simulink model "CEGR_TestBench_10kW_v01_pO2_DQ60"  (R2025b)
settings: Solver=FixedStepDiscrete  StartTime=0.0  StopTime=120  FixedStep=0.1  RelTol=1e-3
InitFcn:
  | modelFile=get_param(bdroot,'FileName'); projectDir=fileparts(fileparts(modelFile)); addpath(fullfile(projectDir,'02_脚本')); prepare_testbench_10kw_v01_model_run(bdroot);
model workspace (MAT data in the model file):
  BenchAirParam_v1 = [96485.33212; 0.031998; 0.0280134; 0.01801528; 112.325; 58.9; 0.8; 0.2095; 0.7905; 16; 2; 0.00428414; 141.325; 58.9; 0.8]
  BenchConditionerParam_v1 = [0.031998; 0.0280134; 0.01801528; 101.325; 58.9; 141.325]
  CompressorParam_v2 = [8.314462618; 0.031998; 0.0280134; 0.01801528; 1.4; 1005; 0.62; 4000; 3000; 4000; 5000; 6000; 7000; 8000; 80; 170; 420; 590; 780; 960; 120; 220; 500; 650; 830; 1030; 160; 300; 580; 690; 890; 1070; 210; 380; 660; 760; 940; 1120; 300; 500; 720; 820; 990; 1160; 450; 590; 760; 880; 1040; 1200; 29; 39.5; 36.5; 40; 44.5; 43.5; 25; 33; 26; 33; 35; 32; 22; 27; 16; 27.5; 28; 25; 16; 18.5; 10.5; 19.5; 20.5; 18; 9; 9; 6; 13; 15; 15; 2.5; 4; 3; 8; 7; 6.5]
  EGRInitialNode_v2 = [0; 0; 0; 0; 56; 133.825; 0]
  EnvParam_v2 = [96485.33212; 0.031998; 0.0280134; 0.01801528; 101.325; 25; 0.5; 0.2095; 0.7905; 16; 2]
  HumidifierParam_v2 = [0.031998; 0.0280134; 0.01801528; 101.325; 55; 0.47854; 0.0983333333333; 0.37998; 0.5825; 9.51831; 11.4663; 0.578752; 40; 5e-05; 1e-09; 0.06; 0.06; 80]
  I_stack_cmd_A = 38
  IntercoolerParam_v2 = [0.031998; 0.0280134; 0.01801528; 101.325; 55; 8]
  P_v2.rootDir = 'E:\Codex\agentwork_pemfc_cEGR_0519\01_自吸方案\01_车载系统_10kW_GZS60_v3'
  P_v2.inputDir = 'E:\Codex\agentwork_pemfc_cEGR_0519\01_自吸方案\01_车载系统_10kW_GZS60_v3\00_输入参数'
  P_v2.modelName = 'CEGR_Vehicle_10kW_GZS60_v03_stage1_pressurefix'
  P_v2.modelFile = 'E:\Codex\agentwork_pemfc_cEGR_0519\01_自吸方案\01_车载系统_10kW_GZS60_v3\01_模型\CEGR_Vehicle_10kW_GZS60_v03_stage1_pressurefix.slx'
  P_v2.calibration_baseline = "stage1_pressurefix_no_egr"
  P_v2.stopTime_s = 120
  P_v2.dt_s = 0.1
  P_v2.R_J_molK = 8.314462618
  P_v2.F_C_mol = 96485.33212
  P_v2.M_O2_kg_mol = 0.031998
  P_v2.M_N2_kg_mol = 0.0280134
  P_v2.M_H2O_kg_mol = 0.01801528
  P_v2.M_H2_kg_mol = 0.00201588
  P_v2.p_amb_kPa = 101.325
  P_v2.T_amb_C = 25
  P_v2.RH_amb = 0.5
  P_v2.xO2_dry = 0.2095
  P_v2.xN2_dry = 0.7905
  P_v2.N_cell = 16
  P_v2.A_cell_cm2 = 380
  P_v2.I_stack_default_A = 120
  P_v2.oxygen_stoich = 2
  P_v2.anode_stoich = 1.35
  P_v2.RH_an_in = 0.3
  P_v2.compressor_dp_kPa = 55
  P_v2.compressor_dT_C = 35
  P_v2.intercooler_T_C = 55
  P_v2.intercooler_dp_kPa = 8
  P_v2.p_cathode_back_kPa = 128
  P_v2.p_anode_back_kPa = 85
  P_v2.p_anode_in_kPa = 140
  P_v2.K_ca_in_kg_s_kPa = 0.0003
  P_v2.hum_NTU_ref = 0.47854
  P_v2.hum_m_ref_kg_s = 0.0983333333333
  P_v2.hum_flow_exp = 0.37998
  P_v2.hum_heat_eff = 0.5825
  P_v2.hum_dry_dp_ref_kPa = 9.51831
  P_v2.hum_wet_dp_ref_kPa = 11.4663
  P_v2.hum_dp_exp = 0.578752
  P_v2.hum_mem_area_m2 = 40
  P_v2.hum_mem_thickness_m = 5e-05
  P_v2.hum_mem_D_eff_m2_s = 1e-09
  P_v2.hum_beta_wet_m_s = 0.06
  P_v2.hum_beta_dry_m_s = 0.06
  P_v2.hum_UA_W_K = 80
  P_v2.V_ca_m3 = 0.0002
  P_v2.V_an_m3 = 0.00015
  P_v2.K_ca_out_kg_s_kPa = 0.00012
  P_v2.K_an_out_kg_s_kPa = 6.67e-06
  P_v2.K_liq_carry_1_s = 0.08
  P_v2.C_stack_J_K = 45000
  P_v2.h_cool_W_K = 836
  P_v2.T_cool_C = 62
  P_v2.h_amb_W_K = 9
  P_v2.coolant_flow_L_min = 6
  P_v2.coolant_rho_kg_L = 1
  P_v2.coolant_cp_J_kgK = 4180
  P_v2.cool_flow_curve_enabled = 1
  P_v2.cool_flow_curve_L_min = [5.5 6 6.5 7.5 9.1 10 11.1 11.5 0 0 0 0 0]
  P_v2.cool_flow_curve_h_W_K = [836 836 905.666666667 1045 1267.93333333 1393.33333333 1546.6 1602.33333333 0 0 0 0 0]
  P_v2.k_mem_water_kg_s = 0.00012
  P_v2.E_nernst_ref_V = 1.229
  P_v2.E_nernst_temp_coeff_V_K = 0.00085
  P_v2.book_theta1 = 0.304017191982
  P_v2.book_theta2 = 2.2530615997e-05
  P_v2.book_theta3 = -2.43220427369e-40
  P_v2.book_theta4 = 6.6267870644e-05
  P_v2.book_theta5 = 0.0455473243079
  P_v2.book_theta6 = 6.57684656899e-05
  P_v2.book_theta7 = -1.52874181623
  P_v2.book_theta8 = 9.63813640803e-05
  P_v2.book_theta9 = 2.42869264824e-06
  P_v2.book_theta10 = 0.00979289103499
  P_v2.membraneThickness_cm = 0.005
  P_v2.thermoneutralVoltage_V = 1.254
  P_v2.LHV_H2_J_mol = 241800
  P_v2.stack_m_act_O2 = 0.65
  P_v2.stack_m_lim_O2 = 1.2
  P_v2.stack_i_lim_ref_A_cm2 = 1.2
  P_v2.stack_lambda_O2_half = 1.2
  P_v2.egr_fraction_default = 0.4
  P_v2.EnvParam = [96485.33212; 0.031998; 0.0280134; 0.01801528; 101.325; 25; 0.5; 0.2095; 0.7905; 16; 2]
  P_v2.CompressorParam = [55; 35]
  P_v2.IntercoolerParam = [0.031998; 0.0280134; 0.01801528; 101.325; 55; 8]
  P_v2.HumidifierParam = [0.031998; 0.0280134; 0.01801528; 101.325; 55; 0.47854; 0.0983333333333; 0.37998; 0.5825; 9.51831; 11.4663; 0.578752; 40; 5e-05; 1e-09; 0.06; 0.06; 80]
  P_v2.StackParam = [8.314462618; 96485.33212; 0.031998; 0.0280134; 0.01801528; 0.00201588; 101.325; 25; 16; 380; 0.0002; 0.00015; 0.00012; 6.67e-06; 128; 85; 0.08; 45000; 836; 62; 9; 1.229; 0.00085; 0.304017191982; 2.2530615997e-05; -2.43220427369e-40; 6.6267870644e-05; 0.005; 9.63813640803e-05; 2.42869264824e-06; 0.00979289103499; 1.254; 1.35; 0.3; 0.1; 0.00012; 140; 0.0003; 0.65; 1.2; 1.2; 1.2; 241800; 6; 1; 5.5; 6; 6.5; 7.5; 9.1; 10; 11.1; 11.5; 0; 0; 0; 0; 0; 836; 836; 905.666666667; 1045; 1267.93333333; 1393.33333333; 1546.6; 1602.33333333; 0; 0; 0; 0; 0; 0.0455473243079; 6.57684656899e-05; -1.52874181623]
  P_v2.egr_initial_node = [0; 0; 0; 0; 25; 101.325; 0]
  P_v2.wet_initial_node = [0; 0; 0; 0; 70; 128; 0]
  P_v2.stack_initial_state = [5.69048472088e-05; 0.000189310998745; 3.20381510039e-05; 0; 1.39815625735e-05; 7.2204543855e-06; 0; 65]
  P_v2.stack_initial_state_audit = [5.69048472088e-05; 0.000189310998745; 3.20381510039e-05; 1.39815625735e-05; 7.2204543855e-06; 65]
  StackInitialStateAudit_v3 = [5.69048472088e-05; 0.000189310998745; 3.20381510039e-05; 1.39815625735e-05; 7.2204543855e-06; 65]
  StackInitialState_v2 = [5.89666776843e-05; 0.000206495047021; 1.97861723777e-05; 1.38831382347e-05; 5.56486098123e-06; 58.9]
  StackParam_v2 = [8.314462618; 96485.33212; 0.031998; 0.0280134; 0.01801528; 0.00201588; 101.325; 25; 16; 380; 0.0002; 0.00015; 0.00012; 6.67e-06; 133.825; 144.725; 0.08; 45000; 1156.46666667; 61.6; 9; 1.229; 0.00085; 0.304017191982; 2.2530615997e-05; -2.43220427369e-40; 6.6267870644e-05; 0.005; 9.63813640803e-05; 2.42869264824e-06; 0.00979289103499; 1.254; 5; 0.3; 0.1; 0.00012; 149.125; 0.000571218666667; 0.65; 1.2; 1.2; 1.2; 241800; 5.5; 1; 6; 6.5; 7.5; 9.1; 10; 11.1; 11.5; 0; 0; 0; 0; 0; 0; 1156.46666667; 1156.46666667; 1285.06756757; 1415.36744186; 1614.22764228; 1614.22764228; 1637.16666667; 0; 0; 0; 0; 0; 0; 0.0455473243079; 6.57684656899e-05; -1.52874181623]
  WetInitialNode_v2 = [0; 0; 0; 0; 70; 128; 0]
  egr_fraction_cmd = 0.25
  egr_initial_node = [0; 0; 0; 0; 25; 101.325; 0]
  stack_initial_state_audit = [5.69048472088e-05; 0.000189310998745; 3.20381510039e-05; 1.39815625735e-05; 7.2204543855e-06; 65]
  wet_initial_node = [0; 0; 0; 0; 70; 128; 0]
settings Model: Creator=ADMIN  LastModifiedBy=92465

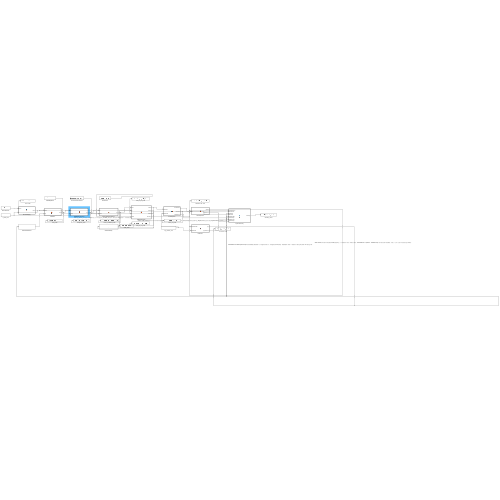
[thumbnail: Simulink's stored preview of the top-level diagram]
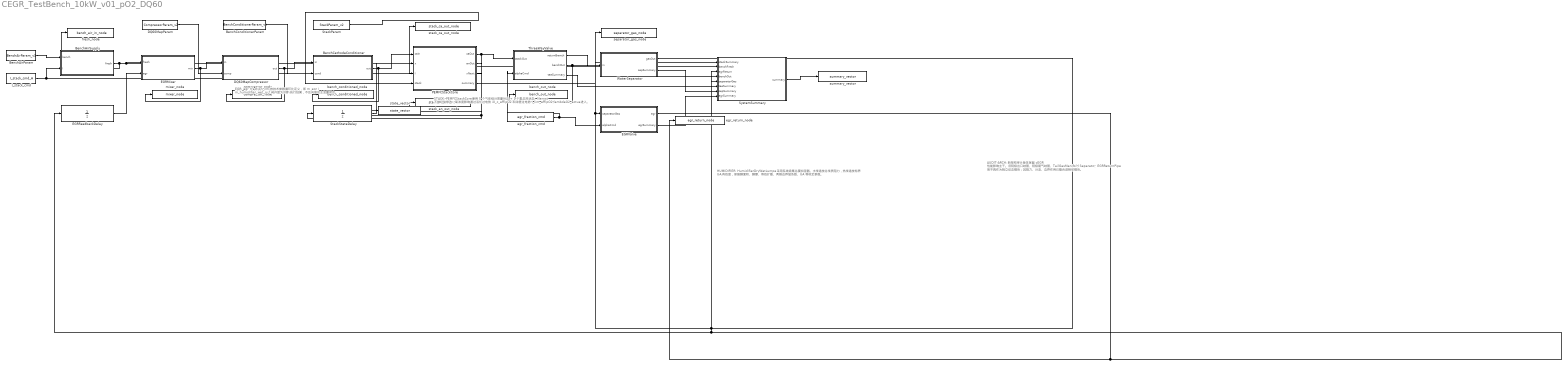
== system CEGR_TestBench_10kW_v01_pO2_DQ60 ==
  note: AUDIT-ARCH: 新架构审计版仅保留 cEGR 性能影响主干。旧阴极出口歧管、阳极尾气歧管、TailGasManifold、Separator、EGRReturnPipe 等不再作为独立动态模块；其阻力、分流、边界作用已整合进相邻模块。
  note: STACK: PEMFCStackCore 使用 5 个气体组分质量状态 + 1 个集总热状态。Nernst 不做经验修改，氧浓度影响通过活化过电势 i0_c_eff(pO2) 和浓差过电势 i_lim_eff(pO2,lambdaO2_actual) 进入。
  note: HUMIDIFIER: HumidifierDryWetLumped 采用系统级集总膜加湿器。水传递按总传质阻力，热传递按有界 UA/有效度，保留膜面积、膜厚、等效扩散、两侧边界层系数、UA 等标定参数。
  note: EGR: egr_fraction_cmd 按技术参数循环比定义，即 m_egr / m_humidifier_wet_out。阀开度为诊断/执行结果，不反向驱动主流量闭合。
  BenchAirParam : Constant  Value=BenchAirParam_v1
  BenchAirSupply : MATLAB Function  TreatAsAtomicUnit=on
  BenchCathodeConditioner : MATLAB Function  TreatAsAtomicUnit=on
  BenchConditionerParam : Constant  Value=BenchConditionerParam_v1
  DQ60MapCompressor : MATLAB Function  TreatAsAtomicUnit=on
  DQ60MapParam : Constant  Value=CompressorParam_v2
  EGRFeedbackDelay : UnitDelay  InitialCondition=EGRInitialNode_v2  SampleTime=-1  HasFrameUpgradeWarning=on
  EGRMixer : MATLAB Function  TreatAsAtomicUnit=on
  EGRValve : MATLAB Function  TreatAsAtomicUnit=on
  I_stack_cmd : Constant  Value=I_stack_cmd_A
  PEMFCStackCore : MATLAB Function  TreatAsAtomicUnit=on
  StackParam : Constant  Value=StackParam_v2
  StackStateDelay : UnitDelay  InitialCondition=StackInitialStateAudit_v3  SampleTime=-1  HasFrameUpgradeWarning=on
  SystemSummary : MATLAB Function  TreatAsAtomicUnit=on
  ThreeWayValve : MATLAB Function  TreatAsAtomicUnit=on
  WaterSeparator : MATLAB Function  TreatAsAtomicUnit=on
  bench_conditioned_node : ToWorkspace  VariableName=bench_conditioned_node  SampleTime=-1
  bench_out_node : ToWorkspace  VariableName=bench_out_node  SampleTime=-1
  compressor_node : ToWorkspace  VariableName=compressor_node  SampleTime=-1
  egr_fraction_cmd : Constant  Value=egr_fraction_cmd
  egr_return_node : ToWorkspace  VariableName=egr_return_node  SampleTime=-1
  fresh_node : ToWorkspace  VariableName=bench_air_in_node  SampleTime=-1
  mixer_node : ToWorkspace  VariableName=mixer_node  SampleTime=-1
  separator_gas_node : ToWorkspace  VariableName=separator_gas_node  SampleTime=-1
  stack_an_out_node : ToWorkspace  VariableName=stack_an_out_node  SampleTime=-1
  stack_ca_out_node : ToWorkspace  VariableName=stack_ca_out_node  SampleTime=-1
  state_vector : ToWorkspace  VariableName=state_vector  SampleTime=-1
  summary_vector : ToWorkspace  VariableName=summary_vector  SampleTime=-1
  wires:
  BenchAirParam/1 -> BenchAirSupply/1(bench)
  I_stack_cmd/1 -> BenchAirSupply/2(I), PEMFCStackCore/3(I)
  BenchAirSupply/1(fresh) -> SystemSummary/2(benchFresh), EGRMixer/1(fresh), fresh_node/1
  EGRFeedbackDelay/1 -> EGRMixer/2(egr)
  EGRMixer/1(mix) -> DQ60MapCompressor/1(in), mixer_node/1
  DQ60MapParam/1 -> DQ60MapCompressor/2(comp)
  DQ60MapCompressor/1(out) -> BenchCathodeConditioner/1(in), compressor_node/1
  BenchConditionerParam/1 -> BenchCathodeConditioner/2(cond)
  BenchCathodeConditioner/1(out) -> bench_conditioned_node/1, PEMFCStackCore/1(caIn)
  StackStateDelay/1 -> PEMFCStackCore/2(x)
  StackParam/1 -> PEMFCStackCore/4(stack)
  PEMFCStackCore/1(caOut) -> ThreeWayValve/1(stackOut), stack_ca_out_node/1
  PEMFCStackCore/2(anOut) -> stack_an_out_node/1
  PEMFCStackCore/3(xNext) -> StackStateDelay/1, state_vector/1
  egr_fraction_cmd/1 -> ThreeWayValve/2(alphaCmd), EGRValve/2(alphaCmd)
  EGRValve/1(egr) -> SystemSummary/3(egrReturn), EGRFeedbackDelay/1, egr_return_node/1
  PEMFCStackCore/4(summary) -> SystemSummary/1(stackSummary)
  EGRValve/2(egrSummary) -> SystemSummary/8(egrSummary)
  SystemSummary/1(summary) -> summary_vector/1
  ThreeWayValve/1(returnBranch) -> WaterSeparator/1(in)
  WaterSeparator/1(gasOut) -> separator_gas_node/1, EGRValve/1(separatorGas), SystemSummary/5(separatorGas)
  ThreeWayValve/2(benchOut) -> bench_out_node/1, SystemSummary/4(benchOut)
  ThreeWayValve/3(teeSummary) -> SystemSummary/6(teeSummary)
  WaterSeparator/2(sepSummary) -> SystemSummary/7(sepSummary)

== matlab function CEGR_TestBench_10kW_v01_pO2_DQ60/EGRMixer ==
  data: fresh input; mix output; egr input
function mix = f(fresh, egr)
%#codegen
% EGR 掺混口径：总进空压机质量流保持新鲜空气基准，回流尾气替代等质量新鲜空气。
mix=zeros(7,1); mf0=max(sum(fresh(1:4)),0); me0=max(sum(egr(1:4)),0); me=min(me0,0.95*mf0); mf=max(mf0-me,0);
wFresh=fresh(1:4)/max(mf0,1e-12); wEgr=egr(1:4)/max(me0,1e-12);
mix(1:4)=mf*wFresh+me*wEgr; mt=max(mf+me,1e-12);
mix(5)=(fresh(5)*mf+egr(5)*me)/mt;
mix(6)=fresh(6); % Compressor inlet pressure follows ambient/suction boundary; EGR pressure is upstream diagnostic only.
mix(7)=double(mix(4)>1e-12);
end

== matlab function CEGR_TestBench_10kW_v01_pO2_DQ60/BenchAirSupply ==
  data: bench input; fresh output; I input
function fresh = f(bench, I)
%#codegen
M_O2=bench(2); M_N2=bench(3); M_H2O=bench(4); p=bench(5); T=bench(6); xO2=bench(8); xN2=bench(9); mTarget=max(bench(12),1e-9);
pStack=bench(13); TStack=bench(14); RHStack=bench(15);
pH2O=min(max(RHStack,0)*sat_kPa(TStack),0.98*pStack); yH2O=min(max(pH2O/max(pStack,1e-6),0),0.98);
yO2=(1-yH2O)*xO2; yN2=(1-yH2O)*xN2;
mO2=yO2*M_O2; mN2=yN2*M_N2; mV=yH2O*M_H2O; s=max(mO2+mN2+mV,1e-12);
fresh=[mTarget*mO2/s; mTarget*mN2/s; mTarget*mV/s; 0; T; p; 0];
end
function p=sat_kPa(T)
Tc=min(max(T,-40),120); p=0.61121*exp((18.678-Tc/234.5)*(Tc/(257.14+Tc)));
end

== matlab function CEGR_TestBench_10kW_v01_pO2_DQ60/DQ60MapCompressor ==
  data: in input; out output; comp input
function out = f(in, comp)
%#codegen
R=comp(1); M_O2=comp(2); M_N2=comp(3); M_H2O=comp(4); gamma=comp(5); cp=comp(6); eta=comp(7); speedRpm=comp(8);
speedGrid=comp(9:14)'; flowGrid=reshape(comp(15:50),6,6); dpGrid=reshape(comp(51:86),6,6);
out=in; T_K=max(in(5)+273.15,150); p_kPa=max(in(6),1);
nDot=max(in(1),0)/M_O2 + max(in(2),0)/M_N2 + max(in(3),0)/M_H2O; mDot=max(sum(in(1:3)),0);
flowLpm=nDot*R*T_K/(p_kPa*1000)*60000;
dpBySpeed=zeros(6,1);
for i=1:6
    q=flowGrid(i,:); d=dpGrid(i,:);
    if flowLpm<=q(1)
        dpBySpeed(i)=d(1);
    elseif flowLpm>=q(end)
        dpBySpeed(i)=d(end);
    else
        dpBySpeed(i)=interp1(q,d,flowLpm,'linear');
    end
end
speed=min(max(speedRpm,speedGrid(1)),speedGrid(end)); dpKPa=interp1(speedGrid,dpBySpeed,speed,'linear');
pOutKPa=p_kPa+max(dpKPa,0); pr=max(pOutKPa/p_kPa,1.0);
dT_K=T_K/max(eta,0.05)*(pr^((gamma-1)/gamma)-1); powerW=mDot*cp*dT_K;
out(5)=T_K+dT_K-273.15; out(6)=pOutKPa; out(7)=double(out(4)>1e-12);
% powerW is local in v01; run scripts recompute diagnostics from logged nodes.
end

== matlab function CEGR_TestBench_10kW_v01_pO2_DQ60/BenchCathodeConditioner ==
  data: in input; out output; cond input
function out = f(in, cond)
%#codegen
M_O2=cond(1); M_N2=cond(2); M_H2O=cond(3); pMin=cond(4); Tout=cond(5);
out=in; out(5)=Tout; out(6)=max(out(6),pMin);
ps=min(sat_kPa(Tout),0.98*out(6)); nDry=max(out(1)/M_O2+out(2)/M_N2,1e-12); mSat=ps*nDry/max(out(6)-ps,1e-6)*M_H2O;
if out(3)>mSat, out(4)=out(4)+out(3)-mSat; out(3)=mSat; end
out(7)=double(out(4)>1e-12);
end
function p=sat_kPa(T)
Tc=min(max(T,-40),120); p=0.61121*exp((18.678-Tc/234.5)*(Tc/(257.14+Tc)));
end

== matlab function CEGR_TestBench_10kW_v01_pO2_DQ60/ThreeWayValve ==
  data: stackOut input; returnBranch output; alphaCmd input; benchOut output; teeSummary output
function [returnBranch, benchOut, teeSummary] = f(stackOut, alphaCmd)
%#codegen
alpha=min(max(alphaCmd,0),0.95);
returnBranch=stackOut; returnBranch(1:4)=alpha*stackOut(1:4); returnBranch(7)=double(returnBranch(4)>1e-12);
benchOut=stackOut; benchOut(1:4)=(1-alpha)*stackOut(1:4); benchOut(7)=double(benchOut(4)>1e-12);
mOutGas=sum(stackOut(1:3)); teeSummary=[alpha; sum(returnBranch(1:3)); sum(benchOut(1:3)); mOutGas; stackOut(4); returnBranch(4); benchOut(4)];
end

== matlab function CEGR_TestBench_10kW_v01_pO2_DQ60/PEMFCStackCore ==
  data: caIn input; caOut output; x input; I input; stack input; anOut output; xNext output; summary output
function [caOut, anOut, xNext, summary] = f(caIn, x, I, stack)
%#codegen
% pcBack is the cathode outlet back-pressure boundary, not a predicted downstream pressure.
R=stack(1); F=stack(2); M_O2=stack(3); M_N2=stack(4); M_H2O=stack(5); M_H2=stack(6); pamb=stack(7); Tamb=stack(8); N=stack(9); A=stack(10);
Vca=stack(11); Van=stack(12); Kca=stack(13); Kan=stack(14); pcBack=stack(15); panBack=stack(16); Cfc=stack(18); hCool=stack(19); Tcool=stack(20); hAmb=stack(21);
Eref=stack(22); Etemp=stack(23); th1=stack(24); th2=stack(25); th3=stack(26); th4=stack(27); deltaCm=stack(28); th8=stack(29); th9=stack(30); th10=stack(31); Vtn=stack(32); anStoich=stack(33); RHAn=stack(34); dt=stack(35); panIn=stack(37); KcaIn=stack(38); th5=stack(72); th6=stack(73); th7=stack(74);
coolantFlow=stack(44);
hCoolEff=hCool; if numel(stack)>=71 && stack(45)>0.5, hCoolEff=interp_hcool_flow(coolantFlow,stack(46:58),stack(59:71),hCool); end
mO2=max(x(1),1e-12); mN2=max(x(2),1e-12); mV=max(x(3),0); mH2=max(x(4),1e-12); mVAn=max(x(5),0); T=x(6); TK=T+273.15;
pO2=mO2/M_O2*R*TK/Vca/1000; pN2=mN2/M_N2*R*TK/Vca/1000; pV=mV/M_H2O*R*TK/Vca/1000; pCa=max(pO2+pN2+pV,pamb);
pVAn=mVAn/M_H2O*R*TK/Van/1000;
mInCmd=sum(caIn(1:3)); mInPressure=KcaIn*max(caIn(6)-pCa,0); mIn=min(mInCmd,mInPressure); wIn=caIn(1:3)/max(mInCmd,1e-12); mO2In=mIn*wIn(1); mN2In=mIn*wIn(2); mVIn=mIn*wIn(3);
mO2React=I*N/(4*F)*M_O2; mH2React=I*N/(2*F)*M_H2; mWater=I*N/(2*F)*M_H2O; lambdaO2=(mO2In/M_O2)/max(I*N/(4*F),1e-12);
ps=sat_kPa(T); aCa=min(max(pV/max(ps,1e-6),0),3); aAn=min(max(pVAn/max(ps,1e-6),0),3); lam=0.5*(lambda_eq(aCa)+lambda_eq(aAn));
A_m2=A*1e-4; nDrag=max(0.0029*lam^2+0.05*lam,0); D=membrane_diff(lam,TK); cCa=pV*1000/(R*TK); cAn=pVAn*1000/(R*TK); mMem=(nDrag*I/F - D*A_m2*N/max(deltaCm*0.01,1e-9)*(cCa-cAn))*M_H2O;
mH2In=anStoich*mH2React; pH2OIn=RHAn*ps; mVAnIn=mH2In*max(pH2OIn,0)/max(panIn-pH2OIn,1e-6)*(M_H2O/M_H2);
mO2Pre=max(mO2+dt*(mO2In-mO2React),1e-12); mN2Pre=max(mN2+dt*mN2In,1e-12); mVPre=max(mV+dt*(mVIn+mWater+mMem),0);
mH2Pre=max(mH2+dt*(mH2In-mH2React),1e-12); mVAnPre=max(mVAn+dt*(mVAnIn-mMem),0);
pO2Pre=mO2Pre/M_O2*R*TK/Vca/1000; pN2Pre=mN2Pre/M_N2*R*TK/Vca/1000; pVPre=mVPre/M_H2O*R*TK/Vca/1000; pCaPre=max(pO2Pre+pN2Pre+pVPre,pamb);
pH2Pre=mH2Pre/M_H2*R*TK/Van/1000; pVAnPre=mVAnPre/M_H2O*R*TK/Van/1000; pAnPre=max(pH2Pre+pVAnPre,pamb);
gasCa=max(mO2Pre+mN2Pre+mVPre,1e-12); wO2=mO2Pre/gasCa; wN2=mN2Pre/gasCa; wV=mVPre/gasCa;
mCaOutRaw=Kca*max(pCaPre-pcBack,0)/(1+Kca*max(pCaPre,1e-6)*dt/gasCa); mCaOut=min(mCaOutRaw,0.95*gasCa/max(dt,1e-9));
gasAn=max(mH2Pre+mVAnPre,1e-12); wH2=mH2Pre/gasAn; wVAn=mVAnPre/gasAn;
mAnOutRaw=Kan*max(pAnPre-panBack,0)/(1+Kan*max(pAnPre,1e-6)*dt/gasAn); mAnOut=min(mAnOutRaw,0.95*gasAn/max(dt,1e-9));
mO2n=max(mO2Pre-dt*wO2*mCaOut,1e-12); mN2n=max(mN2Pre-dt*wN2*mCaOut,1e-12); mVnRaw=max(mVPre-dt*wV*mCaOut,0);
mH2n=max(mH2Pre-dt*wH2*mAnOut,1e-12); mVAnnRaw=max(mVAnPre-dt*wVAn*mAnOut,0);
[mVn,liqDiag]=clip_vapor(mVnRaw,0,mO2n,mN2n,T,pCaPre,stack,0); [mVAnn,liqAnDiag]=clip_vapor(mVAnnRaw,0,mH2n,0,T,pAnPre,stack,1);
phaseCa=(mVnRaw-mVn)/dt; phaseAn=(mVAnnRaw-mVAnn)/dt;
j=max(I/max(A,1e-9),1e-6); E=Eref-Etemp*(TK-298.15)+R*TK/(2*F)*log(max(pH2Pre*1000,1)/101325*sqrt(max(pO2Pre*1000,1)/101325));
CO2=max(1.97e-7*(pO2Pre*1000)*exp(498/TK),1e-12); etaAct=max(th1+th2*TK+th3*TK*log(CO2)+th4*TK*log(max(I,1e-6)),0);
Rm=deltaCm/max(A*(th5*lam+th6)*exp(th7*(1/303.15-1/TK)),1e-12); etaOhm=I*(Rm+th8);
iLim=j; i0Scale=CO2; etaCon=max(th9*exp(min(th10*I,50)),0);
V=E-etaAct-etaOhm-etaCon; Pstack=I*V*N; Qgen=I*N*(Vtn-V); Qcool=hCoolEff*(T-Tcool); Qamb=hAmb*(T-Tamb); Qgas=max(mCaOut+mAnOut,0)*1050*max(T-caIn(5),0); Qnet=Qgen-Qcool-Qamb-Qgas; Tn=T+dt*Qnet/Cfc;
TKn=Tn+273.15; pO2Diag=mO2n/M_O2*R*TKn/Vca/1000; pN2Diag=mN2n/M_N2*R*TKn/Vca/1000; pVDiag=mVn/M_H2O*R*TKn/Vca/1000; pCaDiag=max(pO2Diag+pN2Diag+pVDiag,pamb);
pH2Diag=mH2n/M_H2*R*TKn/Van/1000; pVAnDiag=mVAnn/M_H2O*R*TKn/Van/1000; pAnDiag=max(pH2Diag+pVAnDiag,pamb);
xNext=[mO2n;mN2n;mVn;mH2n;mVAnn;Tn]; caOut=[wO2*mCaOut;wN2*mCaOut;wV*mCaOut;0;Tn+3;pcBack;0]; anOut=[wH2*mAnOut;0;wVAn*mAnOut;0;Tn;panBack;0];
nTot=max(mO2n/M_O2+mN2n/M_N2+mVn/M_H2O,1e-12); xO2=(mO2n/M_O2)/nTot; RH=(mVn/M_H2O*R*(Tn+273.15)/Vca/1000)/max(sat_kPa(Tn),1e-6);
nInTot=max(caIn(1)/M_O2+caIn(2)/M_N2+caIn(3)/M_H2O,1e-12); xO2In=(caIn(1)/M_O2)/nInTot; pO2In=caIn(6)*xO2In; RHIn=(caIn(6)*(caIn(3)/M_H2O)/nInTot)/max(sat_kPa(caIn(5)),1e-6);
resO2=(mO2n-mO2)/dt-(mO2In-wO2*mCaOut-mO2React); resN2=(mN2n-mN2)/dt-(mN2In-wN2*mCaOut);
resH2Ov=(mVn-mV)/dt-(mVIn-wV*mCaOut+mWater+mMem-phaseCa);
resH2=(mH2n-mH2)/dt-(mH2In-wH2*mAnOut-mH2React); resH2OvAn=(mVAnn-mVAn)/dt-(mVAnIn-wVAn*mAnOut-mMem-phaseAn);
maxGasRes=max(abs([resO2,resN2,resH2Ov,resH2,resH2OvAn]));
summary=[I;V;Pstack;pO2Diag;pCaDiag;pH2Diag;pAnDiag;lam;Tn;xO2;RH;mMem;mO2React;mH2React;mWater;mCaOut;mAnOut;Cfc*(Tn-T)/dt-Qnet;pO2In;xO2In;RHIn;Qnet;resO2;resN2;resH2Ov;phaseCa;resH2;resH2OvAn;phaseAn;phaseCa+phaseAn;maxGasRes;Qgen;Qcool;Qamb;Qgas;E;etaAct;etaOhm;etaCon;lambdaO2;mIn;iLim;i0Scale;mVIn;wV*mCaOut;mVAnIn;wVAn*mAnOut;liqDiag+liqAnDiag];
end
function [mv,ml]=clip_vapor(mv0,ml0,mA,mB,T,p,stack,isAnode)
M_O2=stack(3); M_N2=stack(4); M_H2O=stack(5); M_H2=stack(6); MA=M_O2; MB=M_N2; if isAnode>0.5, MA=M_H2; end; ps=min(sat_kPa(T),0.98*p); nDry=max(mA/MA+mB/MB,1e-12); mSat=max(ps*nDry/max(p-ps,1e-6)*M_H2O,0); if mv0>mSat, mv=mSat; ml=ml0+mv0-mSat; else, mv=mv0; ml=ml0; end
end
function p=sat_kPa(T)
Tc=min(max(T,-40),120); p=0.61121*exp((18.678-Tc/234.5)*(Tc/(257.14+Tc)));
end
function lambda=lambda_eq(a)
if a<=1, lambda=0.043+17.81*a-39.85*a^2+36*a^3; else, lambda=14+1.4*(a-1); end
end
function D=membrane_diff(lambda,TK)
if lambda<2, d0=1e-10; elseif lambda<3, d0=1e-10*(1+2*(lambda-2)); elseif lambda<4.5, d0=1e-10*(3-1.167*(lambda-3)); else, d0=1.25e-10; end; D=d0*exp(2416*(1/303-1/max(TK,1)));
end
function h=interp_hcool_flow(flow,bp,hv,hFallback)
n=0; for k=1:numel(bp), if bp(k)>0 && hv(k)>0, n=n+1; end, end; if n<2, h=hFallback; return; end
b=zeros(n,1); v=zeros(n,1); j=0; for k=1:numel(bp), if bp(k)>0 && hv(k)>0, j=j+1; b(j)=bp(k); v(j)=hv(k); end, end
if flow<=b(1), h=v(1); return; end; if flow>=b(n), h=v(n); return; end
h=v(n); for k=1:n-1, if flow>=b(k) && flow<=b(k+1), a=(flow-b(k))/max(b(k+1)-b(k),1e-9); h=v(k)+a*(v(k+1)-v(k)); return; end, end
end

== matlab function CEGR_TestBench_10kW_v01_pO2_DQ60/EGRValve ==
  data: separatorGas input; egr output; alphaCmd input; egrSummary output
function [egr, egrSummary] = f(separatorGas, alphaCmd)
%#codegen
egr=separatorGas; egr(4)=0; egr(7)=0;
mGas=sum(separatorGas(1:3)); egrSummary=[min(max(alphaCmd,0),0.95); mGas; mGas; separatorGas(4)];
end

== matlab function CEGR_TestBench_10kW_v01_pO2_DQ60/WaterSeparator ==
  data: in input; gasOut output; sepSummary output
function [gasOut, sepSummary] = f(in)
%#codegen
M_O2=0.031998; M_N2=0.0280134; M_H2O=0.01801528;
gasOut=in; p=max(in(6),1e-6); T=in(5);
ps=min(sat_kPa(T),0.98*p); nDry=max(in(1)/M_O2+in(2)/M_N2,1e-12); mSat=ps*nDry/max(p-ps,1e-6)*M_H2O;
condensed=max(in(3)-mSat,0); gasOut(3)=in(3)-condensed;
drain=in(4)+condensed; gasOut(4)=0; gasOut(7)=0;
sepSummary=[drain; condensed; in(4); rel_hum(gasOut,M_O2,M_N2,M_H2O); T; p; sum(gasOut(1:3))];
end
function rh=rel_hum(node,M_O2,M_N2,M_H2O)
nV=max(node(3)/M_H2O,0); nt=max(node(1)/M_O2+node(2)/M_N2+nV,1e-12); rh=node(6)*nV/nt/max(sat_kPa(node(5)),1e-6);
end
function p=sat_kPa(T)
Tc=min(max(T,-40),120); p=0.61121*exp((18.678-Tc/234.5)*(Tc/(257.14+Tc)));
end

== matlab function CEGR_TestBench_10kW_v01_pO2_DQ60/SystemSummary ==
  data: stackSummary input; summary output; benchFresh input; egrReturn input; benchOut input; separatorGas input; teeSummary input; sepSummary input; egrSummary input
function summary = f(stackSummary, benchFresh, egrReturn, benchOut, separatorGas, teeSummary, sepSummary, egrSummary)
%#codegen
mStackOut=max(teeSummary(4),1e-12); alphaActual=sum(egrReturn(1:3))/mStackOut;
summary=[stackSummary; sum(benchFresh(1:3)); sum(egrReturn(1:3)); sum(benchOut(1:3)); sum(separatorGas(1:3)); teeSummary; sepSummary; egrSummary; alphaActual; benchFresh(5); benchFresh(6); egrReturn(5); egrReturn(6)];
end
